simulink subsystem "BatteryHV_Custom1_refsub"  (R2026a)
settings: Solver=VariableStepAuto
settings Model: Creator=isaacito  LastModifiedBy=isaacito

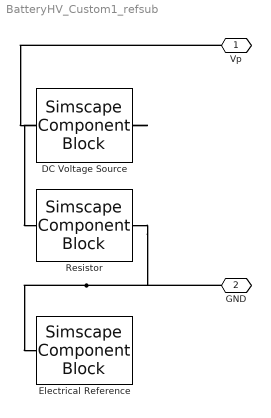
== system BatteryHV_Custom1_refsub ==
  DC Voltage Source : SimscapeComponentBlock  SourceFile=DCVoltageSource  ComponentPath=DCVoltageSource  ComponentVariants="[\"DCVoltageSource\"]"  ComponentVariantNames="[\"DCVoltageSource\"]"  ClassName=DCVoltageSource  SchemaVersion=1  v0=400 V  i_specify=off  i_priority=None  i=0 A  i_nominal_specify=off  i_nominal_value=1  i_nominal_unit=A  v_specify=off  v_priority=None  v=0 V  v_nominal_specify=off  v_nominal_value=1  v_nominal_unit=V
      settings: CopyFcn=simscape.sscblock.internal.componentBlockCallback(gcbh,'COPY')  PreCopyFcn=simscape.sscblock.internal.componentBlockCallback(gcbh,'PRECOPY')  PreDeleteFcn=simscape.sscblock.internal.componentBlockCallback(gcbh,'PREDELETE')
      mask Type: DC Voltage Source
  Electrical Reference : SimscapeComponentBlock  SourceFile=ElectricalReference1  ComponentPath=ElectricalReference1  ComponentVariants="[\"ElectricalReference1\"]"  ComponentVariantNames="[\"ElectricalReference1\"]"  ClassName=ElectricalReference1  SchemaVersion=1  i_specify=off  i_priority=None  i=0 A  i_nominal_specify=off  i_nominal_value=1  i_nominal_unit=A  v_specify=off  v_priority=None  v=0 V  v_nominal_specify=off  v_nominal_value=1  v_nominal_unit=V
      settings: CopyFcn=simscape.sscblock.internal.componentBlockCallback(gcbh,'COPY')  PreCopyFcn=simscape.sscblock.internal.componentBlockCallback(gcbh,'PRECOPY')  PreDeleteFcn=simscape.sscblock.internal.componentBlockCallback(gcbh,'PREDELETE')
      mask Type: Electrical Reference
  Resistor : SimscapeComponentBlock  SourceFile=Resistor  ComponentPath=Resistor  ComponentVariants="[\"Resistor\"]"  ComponentVariantNames="[\"Resistor\"]"  ClassName=Resistor  SchemaVersion=1  R=0.01 Ohm  i_specify=off  i_priority=None  i=0 A  i_nominal_specify=off  i_nominal_value=1  i_nominal_unit=A  v_specify=off  v_priority=None  v=0 V  v_nominal_specify=off  v_nominal_value=1  v_nominal_unit=V
      settings: CopyFcn=simscape.sscblock.internal.componentBlockCallback(gcbh,'COPY')  PreCopyFcn=simscape.sscblock.internal.componentBlockCallback(gcbh,'PRECOPY')  PreDeleteFcn=simscape.sscblock.internal.componentBlockCallback(gcbh,'PREDELETE')
      mask Type: Resistor
  Vp : PMIOPort  Side=Left
  GND : PMIOPort  Port=2  Side=Left
  connections:
  GND/RConn1 -- Electrical Reference/LConn1 -- Resistor/RConn1
  DC Voltage Source/RConn1 -- Resistor/LConn1
  Vp/RConn1 -- DC Voltage Source/LConn1
